simulink model "q3a3576"  (Simulink 7.7)
settings: Solver=ode45  StartTime=0.0  StopTime=10.0  RelTol=1e-3
libraries: simulink x1
settings Model: Creator=Owner  LastModifiedBy=Owner

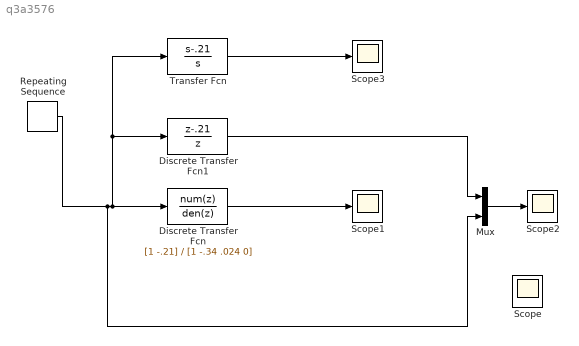
== system q3a3576 ==
  Discrete Transfer Fcn : DiscreteTransferFcn  Numerator=[1 -.21]  Denominator=[1 -.34 .024 0]
  Discrete Transfer Fcn1 : DiscreteTransferFcn  Numerator=[1 -.21]  Denominator=[1 0]
  Mux : Mux  Inputs=2
  Repeating Sequence : simulink/Sources/Repeating Sequence  SystemSampleTime=-1  rep_seq_t=[0:.02:1]  rep_seq_y=[.21.^[1:1:51]]
  Scope{,1..3} (4 alike) : Scope
      Scope1 settings: TimeRange=10  YMin=0  YMax=0.25
      Scope2 settings: SaveName=ScopeData2
      Scope3 settings: SaveName=ScopeData3
  Transfer Fcn : TransferFcn  Numerator=[1 -.21]  Denominator=[1 0]
  wires:
  Repeating Sequence/1 -> Discrete Transfer Fcn/1, Discrete Transfer Fcn1/1, Transfer Fcn/1, Mux/2
  Transfer Fcn/1 -> Scope3/1
  Discrete Transfer Fcn/1 -> Scope1/1
  Discrete Transfer Fcn1/1 -> Mux/1
  Mux/1 -> Scope2/1
